simulink model "VC_v1p1"  (R2022b)
settings: Solver=VariableStepAuto  StartTime=0.0  StopTime=inf  FixedStep=1/100  MaxStep=ts  RelTol=1e-3
InitFcn:
  | init_car
  | init_par
values from neighbouring files (symbols this model uses):
  east0 = EWP(1)    [run_VC_bench.m]
  g = 9.81    [init_car.m]
  north0 = NWP(1)    [run_VC_bench.m]
  NUM_WP = length(NWP)    [run_VC_bench.m]
  psi0 = (pi/180)*HWP(1)    [run_VC_bench.m]
  ts = 1/fs    (= 0.01)    [init_car.m]
  vcg0 = 0    [run_VC_bench.m]
  WPT_MTX = [NWP,EWP,HWP,VWP,KWP,SWP]    [run_VC_bench.m]
undefined symbols (not defined in the file or in its folder): car, EWP, NWP, par, ZWP
libraries: simulink x9, matrix_library x6
(part 2 of 3)

== system VC_v1p1/Chevy Bolt EUV 2023 and GNSS/GNSS measurement/Project vc onto x-y axis ==
  psi (rad) : Inport
  vcg (m/s) : Inport  Port=2
  Product : Product  OutDataTypeStr=double
  Product1 : Product  OutDataTypeStr=double
  Trigonometric Function : Trigonometry  OutputSignalType=real
  Trigonometric Function1 : Trigonometry  Operator=cos  OutputSignalType=real
  vcgx (m/s) : Outport
  vcgy (m/s) : Outport  Port=2
  wires:
  Product/1 -> vcgx (m/s)/1  "vcgx (m/s)"
  Product1/1 -> vcgy (m/s)/1  "vcgy (m/s)"
  psi (rad)/1 -> Trigonometric Function1/1, Trigonometric Function/1
  Trigonometric Function1/1 -> Product/1
  Trigonometric Function/1 -> Product1/2
  vcg (m/s)/1 -> Product1/1, Product/2

== system VC_v1p1/Chevy Bolt EUV 2023 and GNSS/GNSS measurement/Subsystem ==
  note: $a_{lat} = \left( \frac{V_{cg}^2}{R} \right) = \left( \kappa\:V_{cg}^2 \right)$
  vcg (m/s) : Inport
  kappa (1/m) : Inport  Port=2
  multiply : Product
  multiply1 : Product
  alat (m/s/s) : Outport
  wires:
  vcg (m/s)/1 -> multiply/2, multiply/1
  kappa (1/m)/1 -> multiply1/2  "kappa (1/m)"
  multiply/1 -> multiply1/1  "vcg^2 (m^2/s^2)"
  multiply1/1 -> alat (m/s/s)/1  "alat (m/s/s)"

== system VC_v1p1/Chevy Bolt EUV 2023 and GNSS/engine-steer-brake and inertial dynamics/Brake Dynamics ==
  brake_cmd (Nm) : Inport
  torque_cmd (Nm) : Inport  Port=2
  Brake Saturation : Saturate  UpperLimit=car.MAX_BRAKE  LowerLimit=car.MIN_BRAKE  OutDataTypeStr=double
  Compare To Zero : simulink/Logic and Bit Operations/Compare To Zero  relop=>  OutDataTypeStr=boolean
  Compare To Zero1 : simulink/Logic and Bit Operations/Compare To Zero  relop=>=  OutDataTypeStr=boolean
  Logical Operator : Logic  Operator=OR  AllPortsSameDT=off  OutDataTypeStr=boolean
  Resettable Subsystem : Subsystem  TreatAsAtomicUnit=on
  brake dead zone : Subsystem
  brake_fbk (Nm) : Outport
  wires:
  brake_cmd (Nm)/1 -> Compare To Zero1/1, Brake Saturation/1
  Brake Saturation/1 -> Resettable Subsystem/1(In1)
  Resettable Subsystem/1(Out1) -> brake dead zone/1(brake_fbk)
  brake dead zone/1(brake_fbk (Nm)) -> brake_fbk (Nm)/1  "brake_fbk (Nm)"
  torque_cmd (Nm)/1 -> Compare To Zero/1
  Compare To Zero1/1 -> Logical Operator/2
  Compare To Zero/1 -> Logical Operator/1
  Logical Operator/1 -> Resettable Subsystem/Reset

== system VC_v1p1/Chevy Bolt EUV 2023 and GNSS/engine-steer-brake and inertial dynamics/Car Longitudinal Dynamics ==
  note: Note: vcg is the velocity measured at the CG of the car
  Fnet (N) : Inport
  1/ vehicle mass (kg) : Gain  Gain=1/car.MCAR  OutDataTypeStr=double
  Integrator : Integrator  InitialConditionSource=external
  initial vcg (m/s) : Constant  Value=vcg0
  velocity dead zone : Subsystem
  vcg (m/s) : Outport
  along  (m/s/s) : Outport  Port=2
  wires:
  1/ vehicle mass (kg)/1 -> along  (m/s/s)/1, Integrator/1  "acar (m/s/s)"
  Integrator/1 -> velocity dead zone/1(vcg)
  Fnet (N)/1 -> 1/ vehicle mass (kg)/1  "Fnet (N)"
  initial vcg (m/s)/1 -> Integrator/2
  velocity dead zone/1(vcg (m/s)) -> vcg (m/s)/1  "vcg (m/s)"

== system VC_v1p1/Chevy Bolt EUV 2023 and GNSS/engine-steer-brake and inertial dynamics/Engine Torque Dynamics ==
  note: gear: 1=drive, 0=park, -1=reverse
  torque_cmd (Nm) : Inport
  brake_cmd (Nm) : Inport  Port=2
  gear : Inport  Port=3
  Compare To Zero : simulink/Logic and Bit Operations/Compare To Zero  relop=<  OutDataTypeStr=boolean
  Compare To Zero1 : simulink/Logic and Bit Operations/Compare To Zero  relop=<=  OutDataTypeStr=boolean
  Constant : Constant  Value=0
  Constant1 : Constant  Value=0
  Logical Operator : Logic  Operator=OR  AllPortsSameDT=off  OutDataTypeStr=boolean
  Resettable Subsystem : Subsystem  TreatAsAtomicUnit=on
  Torque Saturation : Saturate  UpperLimit=car.MAX_TORQUE  LowerLimit=car.MIN_TORQUE  OutDataTypeStr=double
  do not allow any torque when in park : Switch  Criteria=u2 ~= 0  SaturateOnIntegerOverflow=off  InputSameDT=off
  "do not allow any torque when in park " : Switch  Criteria=u2 ~= 0  SaturateOnIntegerOverflow=off  InputSameDT=off
  torque dead zone : Subsystem
  torque_fbk (Nm) : Outport
  wires:
  gear/1 -> "do not allow any torque when in park "/2, do not allow any torque when in park/2
  torque_cmd (Nm)/1 -> Compare To Zero1/1, do not allow any torque when in park/1
  Constant/1 -> do not allow any torque when in park/3
  do not allow any torque when in park/1 -> Torque Saturation/1
  Constant1/1 -> "do not allow any torque when in park "/3
  "do not allow any torque when in park "/1 -> torque dead zone/1(torque_fbk)
  torque dead zone/1(torque_fbk (Nm)) -> torque_fbk (Nm)/1
  Torque Saturation/1 -> Resettable Subsystem/1(In1)
  Resettable Subsystem/1(Out1) -> "do not allow any torque when in park "/1  "torque_fbk (Nm)"
  brake_cmd (Nm)/1 -> Compare To Zero/1
  Logical Operator/1 -> Resettable Subsystem/Reset
  Compare To Zero/1 -> Logical Operator/1
  Compare To Zero1/1 -> Logical Operator/2

== system VC_v1p1/Chevy Bolt EUV 2023 and GNSS/engine-steer-brake and inertial dynamics/Net Force Applied at CG ==
  torque_fbk (Nm) : Inport
  brake_fbk (Nm) : Inport  Port=2
  Fgrade (N) : Inport  Port=3
  vcg (m/s) : Inport  Port=4
  1 / Tire Radius : Gain  Gain=1 / car.Rtire
  "1 / Tire Radius " : Gain  Gain=1 / car.Rtire
  Bus Creator : BusCreator  Inputs=4
  MATLAB Function : MATLAB Function  TreatAsAtomicUnit=on
  Sum : Sum  Inputs=++-
  To Workspace2 : ToWorkspace  VariableName=forces  SampleTime=ts
  deadzone velocity1 : Constant  Value=car.Vdead  SampleTime=ts
  rolling resistance (Ns/m) : Gain  Gain=car.RRdamp
  Fnet (N) : Outport
  wires:
  vcg (m/s)/1 -> MATLAB Function/3(vcg), rolling resistance (Ns/m)/1
  torque_fbk (Nm)/1 -> 1 / Tire Radius/1
  brake_fbk (Nm)/1 -> "1 / Tire Radius "/1
  1 / Tire Radius/1 -> Sum/2  "Ftorque (N)"
  "1 / Tire Radius "/1 -> MATLAB Function/4(Fbrake)  "Fbrake (N)"
  deadzone velocity1/1 -> MATLAB Function/2(Vdead)
  rolling resistance (Ns/m)/1 -> Bus Creator/4, Sum/3  "Fdamp (N)"
  Sum/1 -> Bus Creator/2, MATLAB Function/1(Fsum)  "Fsum (N)"
  Fgrade (N)/1 -> Bus Creator/1, Sum/1  "Fgrade (N)"
  Bus Creator/1 -> To Workspace2/1
  MATLAB Function/1(Fnet) -> Bus Creator/3, Fnet (N)/1  "Fnet (N)"

== system VC_v1p1/Chevy Bolt EUV 2023 and GNSS/engine-steer-brake and inertial dynamics/Road Grade Force ==
  note: NOTE: Positive grade (pitch) means "pointing uphill", which makes the force due to grade (Fgrade) have a negative value as well as the resulting effective grade torque (Tgrade).
  grade (rad) : Inport
  gear_fbk : Inport  Port=2
  Compare To Zero : simulink/Logic and Bit Operations/Compare To Zero  relop=~=  OutDataTypeStr=boolean
  Constant : Constant  Value=0
  Do not allow grade force when car is in Park : Switch  Criteria=u2 > Threshold  SaturateOnIntegerOverflow=off  InputSameDT=off
  To Workspace2 : ToWorkspace  VariableName=Fgrade  SampleTime=ts
  Trigonometric Function : Trigonometry
  account for direction of force with grade : Gain  Gain=-1
  grade component : Gain  Gain=car.MCAR * g  OutDataTypeStr=double
  pitch (rad) : Outport
  Fgrade (N) : Outport  Port=2
  wires:
  grade component/1 -> account for direction of force with grade/1
  grade (rad)/1 -> pitch (rad)/1, Trigonometric Function/1  "assume no pitch dynamics so pitch = grade"
  Trigonometric Function/1 -> grade component/1
  account for direction of force with grade/1 -> Do not allow grade force when car is in Park/1
  Compare To Zero/1 -> Do not allow grade force when car is in Park/2
  gear_fbk/1 -> Compare To Zero/1
  Constant/1 -> Do not allow grade force when car is in Park/3
  Do not allow grade force when car is in Park/1 -> To Workspace2/1, Fgrade (N)/1  "Fgrade (Nm)"

== system VC_v1p1/Chevy Bolt EUV 2023 and GNSS/engine-steer-brake and inertial dynamics/Steering Dynamics ==
  steer_cmd (deg) : Inport
  Gain conversion from steering angle (deg) to front wheel angle (deg) : Gain  Gain=car.STEER_RATIO
  Steering Saturation : Saturate  UpperLimit=car.MAX_STEER  LowerLimit=car.MIN_STEER  OutDataTypeStr=double
  deg-to-rad : Gain  Gain=pi/180
  second-order low-pass steer model : TransferFcn  Numerator=car.STEER_NUMS  Denominator=car.STEER_DENS
  steer dead zone : Subsystem
  delta (rad) : Outport
  steer_fbk (deg) : Outport  Port=2
  wires:
  Steering Saturation/1 -> second-order low-pass steer model/1
  steer_cmd (deg)/1 -> Steering Saturation/1
  Gain conversion from steering angle (deg) to front wheel angle (deg)/1 -> deg-to-rad/1  "front wheel  angle (deg)"
  deg-to-rad/1 -> delta (rad)/1
  second-order low-pass steer model/1 -> steer dead zone/1(steer)
  steer dead zone/1(steer (deg)) -> steer_fbk (deg)/1, Gain conversion from steering angle (deg) to front wheel angle (deg)/1  "actual steering wheel angle (deg)"

== system VC_v1p1/Chevy Bolt EUV 2023 and GNSS/kinematic Bicycle model/CG to Rear Coordinate Transformation ==
  pose_cg : Inport
  beta : Inport  Port=2
  Bus Creator1 : BusCreator  Inputs=4
  Bus Selector : BusSelector  OutputSignals=eastcg (m),psi (rad),northcg (m),vcg (m/s)
  Product4 : Product
  Sum7 : Sum  Inputs=+-|
  Sum8 : Sum  Inputs=|-+
  Trigonometric Function5 : Trigonometry  Operator=cos  OutputSignalType=real
  Trigonometric Function6 : Trigonometry  OutputSignalType=real
  Trigonometric Function7 : Trigonometry  Operator=cos  OutputSignalType=real
  cg to rear wheel (m) : Gain  Gain=car.LR
  cg to rear wheel (m)2 : Gain  Gain=car.LR
  pose_rear : Outport
  wires:
  Trigonometric Function6/1 -> cg to rear wheel (m)/1
  Bus Selector/1 -> Sum7/1  "<eastcg (m)>"
  cg to rear wheel (m)/1 -> Sum7/2
  Bus Selector/2 -> Trigonometric Function6/1, Bus Creator1/3, Trigonometric Function5/1  "<psi (rad)>"
  Trigonometric Function5/1 -> cg to rear wheel (m)2/1
  Sum8/1 -> Bus Creator1/2  "northr (m)"
  cg to rear wheel (m)2/1 -> Sum8/1
  Bus Creator1/1 -> pose_rear/1
  beta/1 -> Trigonometric Function7/1
  pose_cg/1 -> Bus Selector/1
  Sum7/1 -> Bus Creator1/1  "eastr (m)"
  Bus Selector/3 -> Sum8/2  "<northcg (m)>"
  Trigonometric Function7/1 -> Product4/2
  Bus Selector/4 -> Product4/1  "<vcg (m/s)>"
  Product4/1 -> Bus Creator1/4  "vr (m/s)"

== system VC_v1p1/Chevy Bolt EUV 2023 and GNSS/kinematic Bicycle model/Vehicle Slip Angle (direction of CG) ==
  note: Curvature: $\kappa = \left( \frac{1}{radius\:of\:curvature} \right)$
  note: Equation 2.7, pg. 23, Rajamani
  note: Equation 2.13, pg. 24, Rajamani
  note: $\beta$ = slip angle of vehicle [radians]
  delta (rad) : Inport
  Divide : Product  Inputs=**/
  Trigonometric Function1 : Trigonometry  Operator=cos  OutputSignalType=real
  Trigonometric Function2 : Trigonometry  Operator=atan2  OutputSignalType=real
  Trigonometric Function3 : Trigonometry  Operator=tan  OutputSignalType=real
  cg to rear wheel (m) : Gain  Gain=car.LR
  wheelbase (m) : Constant  Value=car.LF+car.LR
  "wheelbase (m) " : Constant  Value=car.LF+car.LR
  beta (rad) : Outport
  kappa (1/m) : Outport  Port=2
  wires:
  wheelbase (m)/1 -> Trigonometric Function2/2
  Trigonometric Function2/1 -> Trigonometric Function1/1, beta (rad)/1  "beta"
  Trigonometric Function3/1 -> Divide/2, cg to rear wheel (m)/1  "tan(delta)"
  delta (rad)/1 -> Trigonometric Function3/1
  cg to rear wheel (m)/1 -> Trigonometric Function2/1
  Trigonometric Function1/1 -> Divide/1
  "wheelbase (m) "/1 -> Divide/3
  Divide/1 -> kappa (1/m)/1  "1/R"

== system VC_v1p1/Vehicle_Controller/Data Registers/load new parameter vector ==
  mode_select : Inport
  par_vector : Inport  Port=2
  Subsystem : Subsystem
  edge detector : Subsystem
  par_bus_out : Outport
  wires:
  mode_select/1 -> edge detector/1(in)
  par_vector/1 -> Subsystem/1(par_vector)
  Subsystem/1(par_bus) -> par_bus_out/1
  edge detector/1(out) -> Subsystem/Enable

== system VC_v1p1/Vehicle_Controller/Data Registers/load new waypoint matrix ==
  new_wpts : Inport
  num_wp : Inport  Port=2
  wpt_mtx : Inport  Port=3
  Data Type Conversion : DataTypeConversion  OutDataTypeStr=double  SaturateOnIntegerOverflow=off  RndMeth=Floor
  Subsystem : Subsystem
  edge detector : Subsystem
  wpt_status_change : Outport
  wpt_bus_out : Outport  Port=2
  wires:
  wpt_mtx/1 -> Subsystem/2(WPT_MTX)
  new_wpts/1 -> edge detector/1(in)
  edge detector/1(out) -> Data Type Conversion/1, Subsystem/Enable
  Data Type Conversion/1 -> wpt_status_change/1
  Subsystem/1(WPT_BUS) -> wpt_bus_out/1
  num_wp/1 -> Subsystem/1(NUM_WP)

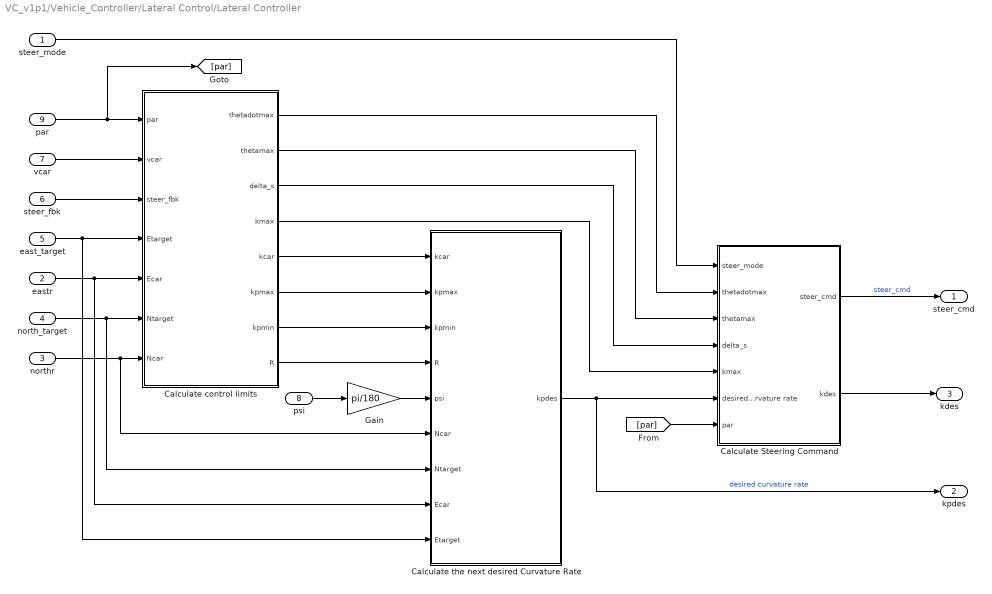
== system VC_v1p1/Vehicle_Controller/Lateral Control/Lateral Controller ==
  steer_mode : Inport
  eastr : Inport  Port=2
  northr : Inport  Port=3
  north_target : Inport  Port=4
  east_target : Inport  Port=5
  steer_fbk : Inport  Port=6
  vcar : Inport  Port=7
  psi : Inport  Port=8
  par : Inport  Port=9
  Calculate Steering Command : Subsystem
  Calculate control limits : Subsystem
  Calculate the next desired Curvature Rate : MATLAB Function  TreatAsAtomicUnit=on  SystemSampleTime=ts
  Gain : Gain  Gain=pi/180
  steer_cmd : Outport
  kpdes : Outport  Port=2
  kdes : Outport  Port=3
  wires:
  par/1 -> [par], Calculate control limits/1(par)
  psi/1 -> Gain/1
  vcar/1 -> Calculate control limits/2(vcar)
  steer_fbk/1 -> Calculate control limits/3(steer_fbk)
  Calculate control limits/5(kcar) -> Calculate the next desired Curvature Rate/1(kcar)
  Calculate control limits/6(kpmax) -> Calculate the next desired Curvature Rate/2(kpmax)
  Calculate control limits/7(kpmin) -> Calculate the next desired Curvature Rate/3(kpmin)
  Calculate control limits/8(R) -> Calculate the next desired Curvature Rate/4(R)
  east_target/1 -> Calculate the next desired Curvature Rate/9(Etarget), Calculate control limits/4(Etarget)
  eastr/1 -> Calculate the next desired Curvature Rate/8(Ecar), Calculate control limits/5(Ecar)
  north_target/1 -> Calculate the next desired Curvature Rate/7(Ntarget), Calculate control limits/6(Ntarget)
  northr/1 -> Calculate the next desired Curvature Rate/6(Ncar), Calculate control limits/7(Ncar)
  steer_mode/1 -> Calculate Steering Command/1(steer_mode)
  Calculate control limits/1(thetadotmax) -> Calculate Steering Command/2(thetadotmax)
  Calculate control limits/2(thetamax) -> Calculate Steering Command/3(thetamax)
  Calculate control limits/3(delta_s) -> Calculate Steering Command/4(delta_s)
  Calculate control limits/4(kmax) -> Calculate Steering Command/5(kmax)
  Calculate the next desired Curvature Rate/1(kpdes) -> kpdes/1, Calculate Steering Command/6(desired curvature rate)  "desired curvature rate"
  [par] -> Calculate Steering Command/7(par)
  Calculate Steering Command/1(steer_cmd) -> steer_cmd/1  "steer_cmd"
  Gain/1 -> Calculate the next desired Curvature Rate/5(psi)
  Calculate Steering Command/2(kdes) -> kdes/1

== system VC_v1p1/Vehicle_Controller/Longitudinal Control/Longitudinal Controller ==
  speed_mode : Inport
  vref : Inport  Port=2
  vcar : Inport  Port=3
  alat : Inport  Port=4
  along : Inport  Port=5
  pitch : Inport  Port=6
  par : Inport  Port=7
  Speed Controller : Subsystem
  velocity feedback pre-processor : Subsystem
  torque_cmd : Outport
  brake_cmd : Outport  Port=2
  vdes : Outport  Port=3
  car_is_stopped : Outport  Port=4
  wires:
  velocity feedback pre-processor/3(verror) -> Speed Controller/2(verror)
  speed_mode/1 -> velocity feedback pre-processor/1(speed_mode), Speed Controller/1(speed_mode)
  par/1 -> Speed Controller/4(par), velocity feedback pre-processor/6(par)
  alat/1 -> velocity feedback pre-processor/4(alat)
  vref/1 -> velocity feedback pre-processor/2(vref)
  velocity feedback pre-processor/1(vdes) -> vdes/1
  vcar/1 -> velocity feedback pre-processor/3(vcar)
  along/1 -> velocity feedback pre-processor/5(along)
  pitch/1 -> Speed Controller/3(pitch)
  Speed Controller/1(torque_cmd) -> torque_cmd/1
  Speed Controller/2(brake_cmd) -> brake_cmd/1
  velocity feedback pre-processor/2(car_is_stopped) -> car_is_stopped/1

== system VC_v1p1/Vehicle_Controller/Pack Data Log Message/Estimate Jerk ==
  Bus Selector : BusSelector  OutputSignals=ts
  Jerk Estimation Filter : MATLAB Function  TreatAsAtomicUnit=on  SystemSampleTime=ts
  jlat (m/s/s/s) : Outport
  jlong (m/s/s/s) : Outport  Port=2
  wires:
  Jerk Estimation Filter/1(jlat) -> jlat (m/s/s/s)/1  "jlat (m/s/s/s)"
  Jerk Estimation Filter/2(jlong) -> jlong (m/s/s/s)/1  "jlong (m/s/s/s)"
  [alat] -> Jerk Estimation Filter/2(alat)
  [along] -> Jerk Estimation Filter/3(along)
  [mode_select] -> Jerk Estimation Filter/1(mode_select)
  [par_bus] -> Bus Selector/1
  Bus Selector/1 -> Jerk Estimation Filter/4(ts)  "<ts>"

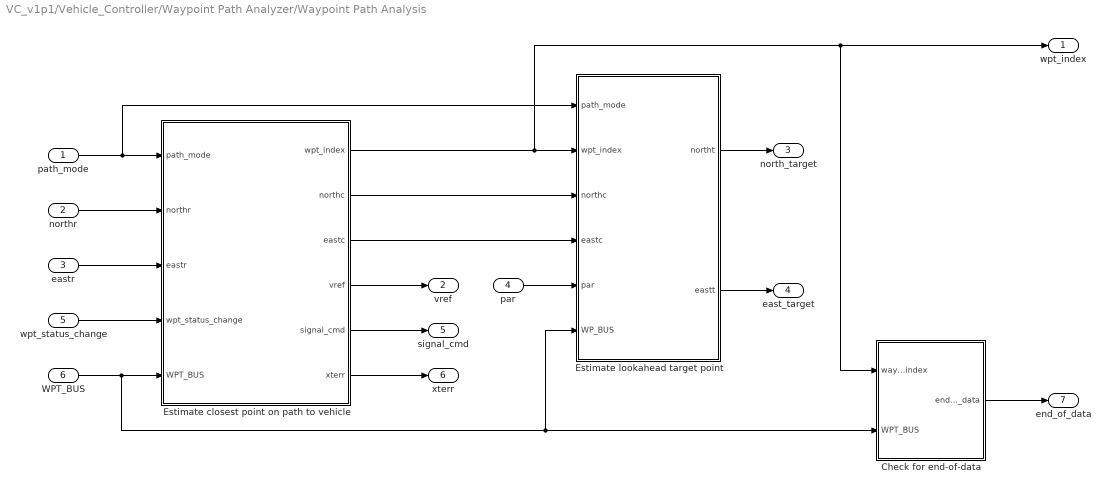
== system VC_v1p1/Vehicle_Controller/Waypoint Path Analyzer/Waypoint Path Analysis ==
  path_mode : Inport
  northr : Inport  Port=2
  eastr : Inport  Port=3
  par : Inport  Port=4
  wpt_status_change : Inport  Port=5
  WPT_BUS : Inport  Port=6
  Check for end-of-data : Subsystem
  Estimate closest point on path to vehicle : Subsystem
  Estimate lookahead target point : Subsystem
  wpt_index : Outport
  vref : Outport  Port=2
  north_target : Outport  Port=3
  east_target : Outport  Port=4
  signal_cmd : Outport  Port=5
  xterr : Outport  Port=6
  end_of_data : Outport  Port=7
  wires:
  path_mode/1 -> Estimate lookahead target point/1(path_mode), Estimate closest point on path to vehicle/1(path_mode)
  Estimate closest point on path to vehicle/2(northc) -> Estimate lookahead target point/3(northc)
  Estimate closest point on path to vehicle/3(eastc) -> Estimate lookahead target point/4(eastc)
  Estimate closest point on path to vehicle/1(wpt_index) -> Check for end-of-data/1(waypoint_index), wpt_index/1, Estimate lookahead target point/2(wpt_index)
  wpt_status_change/1 -> Estimate closest point on path to vehicle/4(wpt_status_change)
  WPT_BUS/1 -> Estimate lookahead target point/6(WP_BUS), Check for end-of-data/2(WPT_BUS), Estimate closest point on path to vehicle/5(WPT_BUS)
  par/1 -> Estimate lookahead target point/5(par)
  Estimate lookahead target point/1(northt) -> north_target/1
  Estimate lookahead target point/2(eastt) -> east_target/1
  Estimate closest point on path to vehicle/4(vref) -> vref/1
  Estimate closest point on path to vehicle/5(signal_cmd) -> signal_cmd/1
  Estimate closest point on path to vehicle/6(xterr) -> xterr/1
  Check for end-of-data/1(end_of_data) -> end_of_data/1
  northr/1 -> Estimate closest point on path to vehicle/2(northr)
  eastr/1 -> Estimate closest point on path to vehicle/3(eastr)

== system VC_v1p1/Chevy Bolt EUV 2023 and GNSS/engine-steer-brake and inertial dynamics/Brake Dynamics/Resettable Subsystem ==
  In1 : Inport
  Reset : ResetPort  DisableCoverage=on
  second-order low-pass brake model : TransferFcn  Numerator=car.BRAKE_NUMS  Denominator=car.BRAKE_DENS
  Out1 : Outport
  wires:
  In1/1 -> second-order low-pass brake model/1
  second-order low-pass brake model/1 -> Out1/1  "brake_fbk (Nm)"

== system VC_v1p1/Chevy Bolt EUV 2023 and GNSS/engine-steer-brake and inertial dynamics/Brake Dynamics/brake dead zone ==
  brake_fbk : Inport
  Abs : Abs  SaturateOnIntegerOverflow=off
  Compare To Constant : simulink/Logic and Bit Operations/Compare To Constant  relop=>  const=car.Tdead  OutDataTypeStr=boolean
  Constant2 : Constant  Value=0
  Zero output signal when in dead zone : Switch  Criteria=u2 > Threshold  SaturateOnIntegerOverflow=off  InputSameDT=off
  brake_fbk (Nm) : Outport
  wires:
  brake_fbk/1 -> Abs/1, Zero output signal when in dead zone/1
  Abs/1 -> Compare To Constant/1
  Zero output signal when in dead zone/1 -> brake_fbk (Nm)/1  "brake_fbk (Nm)"
  Compare To Constant/1 -> Zero output signal when in dead zone/2
  Constant2/1 -> Zero output signal when in dead zone/3

== system VC_v1p1/Chevy Bolt EUV 2023 and GNSS/engine-steer-brake and inertial dynamics/Car Longitudinal Dynamics/velocity dead zone ==
  vcg : Inport
  Abs : Abs  SaturateOnIntegerOverflow=off
  Compare To Constant : simulink/Logic and Bit Operations/Compare To Constant  relop=>  const=car.Vdead  OutDataTypeStr=boolean
  Constant2 : Constant  Value=0
  Zero output signal when in dead zone : Switch  Criteria=u2 > Threshold  SaturateOnIntegerOverflow=off  InputSameDT=off
  vcg (m/s) : Outport
  wires:
  vcg/1 -> Abs/1, Zero output signal when in dead zone/1
  Abs/1 -> Compare To Constant/1
  Zero output signal when in dead zone/1 -> vcg (m/s)/1  "vcg (m/s)"
  Compare To Constant/1 -> Zero output signal when in dead zone/2
  Constant2/1 -> Zero output signal when in dead zone/3

== system VC_v1p1/Chevy Bolt EUV 2023 and GNSS/engine-steer-brake and inertial dynamics/Engine Torque Dynamics/Resettable Subsystem ==
  In1 : Inport
  Reset : ResetPort  DisableCoverage=on
  second-order low-pass torque model : TransferFcn  Numerator=car.TORQUE_NUMS  Denominator=car.TORQUE_DENS
  Out1 : Outport
  wires:
  In1/1 -> second-order low-pass torque model/1
  second-order low-pass torque model/1 -> Out1/1  "torque_fbk (Nm)"

== system VC_v1p1/Chevy Bolt EUV 2023 and GNSS/engine-steer-brake and inertial dynamics/Engine Torque Dynamics/torque dead zone ==
  torque_fbk : Inport
  Abs : Abs  SaturateOnIntegerOverflow=off
  Compare To Constant : simulink/Logic and Bit Operations/Compare To Constant  relop=>  const=car.Tdead  OutDataTypeStr=boolean
  Constant2 : Constant  Value=0
  Zero output signal when in dead zone : Switch  Criteria=u2 > Threshold  SaturateOnIntegerOverflow=off  InputSameDT=off
  torque_fbk (Nm) : Outport
  wires:
  torque_fbk/1 -> Abs/1, Zero output signal when in dead zone/1
  Abs/1 -> Compare To Constant/1
  Zero output signal when in dead zone/1 -> torque_fbk (Nm)/1  "torque_fbk (Nm)"
  Compare To Constant/1 -> Zero output signal when in dead zone/2
  Constant2/1 -> Zero output signal when in dead zone/3

== system VC_v1p1/Chevy Bolt EUV 2023 and GNSS/engine-steer-brake and inertial dynamics/Steering Dynamics/steer dead zone ==
  steer : Inport
  Abs : Abs  SaturateOnIntegerOverflow=off
  Compare To Constant : simulink/Logic and Bit Operations/Compare To Constant  relop=>  const=0.5  OutDataTypeStr=boolean
  Constant2 : Constant  Value=0
  Zero output signal when in dead zone : Switch  Criteria=u2 > Threshold  SaturateOnIntegerOverflow=off  InputSameDT=off
  steer (deg) : Outport
  wires:
  steer/1 -> Abs/1, Zero output signal when in dead zone/1
  Abs/1 -> Compare To Constant/1
  Zero output signal when in dead zone/1 -> steer (deg)/1  "steer (deg)"
  Compare To Constant/1 -> Zero output signal when in dead zone/2
  Constant2/1 -> Zero output signal when in dead zone/3

== system VC_v1p1/Vehicle_Controller/Data Registers/load new parameter vector/Subsystem ==
  note: Initialize par_bus with a default vcctor of values. Whenever this subsystem is enabled, a new par_vector is pushed into the par_bus.
      |
      | The output values stored in par_bus are latched when this subsystem is disabled.
  par_vector : Inport
  Enable : EnablePort  ShowOutputPort=on
  Bus Creator : BusCreator  Inputs=32
  Demux : Demux  Outputs=32
  Initial Control Parameters : Constant  Value=par  SampleTime=ts
  Switch : Switch  Criteria=u2 > Threshold  SaturateOnIntegerOverflow=off  InputSameDT=off
  par_bus : Outport
  wires:
  Demux/26 -> Bus Creator/26  "min_lookahead"
  Demux/29 -> Bus Creator/29  "wT"
  Demux/12 -> Bus Creator/12  "min_steer"
  Demux/1 -> Bus Creator/1  "ts"
  Demux/32 -> Bus Creator/32  "zB"
  Demux/27 -> Bus Creator/27  "lookahead_ratelimit"
  Demux/10 -> Bus Creator/10  "max_alat"
  Demux/31 -> Bus Creator/31  "wB"
  Demux/14 -> Bus Creator/14  "kp_speed"
  Demux/24 -> Bus Creator/24  "fbreak_vref"
  Demux/7 -> Bus Creator/7  "max_delta_brake"
  Demux/21 -> Bus Creator/21  "zz_lead"
  Demux/25 -> Bus Creator/25  "max_lookahead"
  Demux/13 -> Bus Creator/13  "max_delta_steer"
  Demux/17 -> Bus Creator/17  "fbreak_diff"
  Demux/8 -> Bus Creator/8  "max_speed"
  Demux/18 -> Bus Creator/18  "kff_gain"
  Demux/20 -> Bus Creator/20  "fz_lead"
  Demux/28 -> Bus Creator/28  "vdead"
  Demux/15 -> Bus Creator/15  "ki_speed"
  Demux/22 -> Bus Creator/22  "fp_lead"
  Demux/3 -> Bus Creator/3  "min_drv_torque"
  Demux/30 -> Bus Creator/30  "zT"
  Demux/16 -> Bus Creator/16  "kd_speed"
  Demux/9 -> Bus Creator/9  "min_speed"
  Demux/23 -> Bus Creator/23  "kappa2theta"
  Bus Creator/1 -> par_bus/1
  Demux/19 -> Bus Creator/19  "fbreak_fflpf"
  Demux/6 -> Bus Creator/6  "max_delta_torque"
  Demux/4 -> Bus Creator/4  "max_brk_torque"
  Demux/11 -> Bus Creator/11  "max_steer"
  Demux/5 -> Bus Creator/5  "min_brk_torque"
  Demux/2 -> Bus Creator/2  "max_drv_torque"
  par_vector/1 -> Switch/1
  Enable/1 -> Switch/2
  Initial Control Parameters/1 -> Switch/3
  Switch/1 -> Demux/1

== system VC_v1p1/Vehicle_Controller/Data Registers/load new parameter vector/edge detector ==
  note: edge detector
  in : Inport
  Relational Operator : RelationalOperator  Operator=~=  OutDataTypeStr=boolean  RndMeth=Simplest  InputSameDT=off
  previous in : UnitDelay  InitialCondition=3  SampleTime=ts  HasFrameUpgradeWarning=on
  out : Outport
  wires:
  in/1 -> Relational Operator/1, previous in/1
  previous in/1 -> Relational Operator/2
  Relational Operator/1 -> out/1

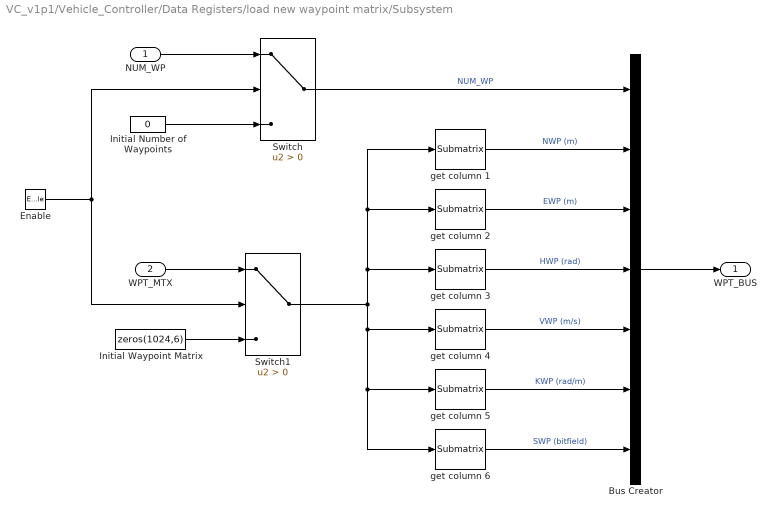
== system VC_v1p1/Vehicle_Controller/Data Registers/load new waypoint matrix/Subsystem ==
  NUM_WP : Inport
  WPT_MTX : Inport  Port=2
  Enable : EnablePort  ShowOutputPort=on
  Bus Creator : BusCreator  Inputs=7
  Initial Waypoint Matrix : Constant  Value=zeros(1024,6)  SampleTime=ts
  "Initial Number of Waypoints   " : Constant  Value=0  SampleTime=ts
  Switch : Switch  Criteria=u2 > Threshold  SaturateOnIntegerOverflow=off  InputSameDT=off
  Switch1 : Switch  Criteria=u2 > Threshold  SaturateOnIntegerOverflow=off  InputSameDT=off
  get column 1 : matrix_library/Submatrix  RowSpan=All rows  RowStartMode=First  RowStartIndex=1  RowEndMode=Last  RowEndIndex=1  ColSpan=One column  ColStartMode=Index  ColStartIndex=1  ColEndMode=Last  ColEndIndex=1
  get column 2 : matrix_library/Submatrix  RowSpan=All rows  RowStartMode=First  RowStartIndex=1  RowEndMode=Last  RowEndIndex=1  ColSpan=One column  ColStartMode=Index  ColStartIndex=2  ColEndMode=Last  ColEndIndex=1
  get column 3 : matrix_library/Submatrix  RowSpan=All rows  RowStartMode=First  RowStartIndex=1  RowEndMode=Last  RowEndIndex=1  ColSpan=One column  ColStartMode=Index  ColStartIndex=3  ColEndMode=Last  ColEndIndex=1
  get column 4 : matrix_library/Submatrix  RowSpan=All rows  RowStartMode=First  RowStartIndex=1  RowEndMode=Last  RowEndIndex=1  ColSpan=One column  ColStartMode=Index  ColStartIndex=4  ColEndMode=Last  ColEndIndex=1
  get column 5 : matrix_library/Submatrix  RowSpan=All rows  RowStartMode=First  RowStartIndex=1  RowEndMode=Last  RowEndIndex=1  ColSpan=One column  ColStartMode=Index  ColStartIndex=5  ColEndMode=Last  ColEndIndex=1
  get column 6 : matrix_library/Submatrix  RowSpan=All rows  RowStartMode=First  RowStartIndex=1  RowEndMode=Last  RowEndIndex=1  ColSpan=One column  ColStartMode=Index  ColStartIndex=6  ColEndMode=Last  ColEndIndex=1
  WPT_BUS : Outport
  wires:
  Bus Creator/1 -> WPT_BUS/1
  get column 4/1 -> Bus Creator/5  "VWP (m/s)"
  get column 5/1 -> Bus Creator/6  "KWP (rad/m)"
  get column 1/1 -> Bus Creator/2  "NWP (m)"
  get column 3/1 -> Bus Creator/4  "HWP (rad)"
  get column 2/1 -> Bus Creator/3  "EWP (m)"
  get column 6/1 -> Bus Creator/7  "SWP (bitfield)"
  Switch/1 -> Bus Creator/1  "NUM_WP"
  NUM_WP/1 -> Switch/1
  WPT_MTX/1 -> Switch1/1
  Switch1/1 -> get column 6/1, get column 5/1, get column 4/1, get column 3/1, get column 2/1, get column 1/1
  Enable/1 -> Switch/2, Switch1/2
  "Initial Number of Waypoints   "/1 -> Switch/3
  Initial Waypoint Matrix/1 -> Switch1/3

== system VC_v1p1/Vehicle_Controller/Data Registers/load new waypoint matrix/edge detector ==
  note: edge detector
  in : Inport
  Relational Operator : RelationalOperator  Operator=~=  OutDataTypeStr=boolean  RndMeth=Simplest  InputSameDT=off
  previous in : UnitDelay  SampleTime=ts  HasFrameUpgradeWarning=on
  out : Outport
  wires:
  in/1 -> Relational Operator/1, previous in/1
  previous in/1 -> Relational Operator/2
  Relational Operator/1 -> out/1

== system VC_v1p1/Vehicle_Controller/Lateral Control/Lateral Controller/Calculate Steering Command ==
  steer_mode : Inport
  thetadotmax : Inport  Port=2
  thetamax : Inport  Port=3
  delta_s : Inport  Port=4
  kmax : Inport  Port=5
  desired curvature rate : Inport  Port=6
  par : Inport  Port=7
  Bus Selector1 : BusSelector  OutputSignals=kappa2theta,ts,max_steer,min_steer,max_delta_steer
  Bus Selector2 : BusSelector  OutputSignals=ts,fz_lead,zz_lead,fp_lead
  Integrate Curvature Rate and compute next Steering Command : MATLAB Function  TreatAsAtomicUnit=on  SystemSampleTime=ts
  MATLAB Function : MATLAB Function  TreatAsAtomicUnit=on  SystemSampleTime=ts
  steer_cmd : Outport
  kdes : Outport  Port=2
  wires:
  desired curvature rate/1 -> Integrate Curvature Rate and compute next Steering Command/6(kpdes)
  thetadotmax/1 -> Integrate Curvature Rate and compute next Steering Command/2(thetadotmax)
  Bus Selector1/1 -> Integrate Curvature Rate and compute next Steering Command/7(kappa2theta)  "<kappa2theta>"
  delta_s/1 -> Integrate Curvature Rate and compute next Steering Command/4(delta_s)
  steer_mode/1 -> MATLAB Function/1(steer_mode), Integrate Curvature Rate and compute next Steering Command/1(steer_mode)
  par/1 -> Bus Selector2/1, Bus Selector1/1
  kmax/1 -> Integrate Curvature Rate and compute next Steering Command/5(kmax)
  Bus Selector1/3 -> Integrate Curvature Rate and compute next Steering Command/9(max_steer)  "<max_steer>"
  thetamax/1 -> Integrate Curvature Rate and compute next Steering Command/3(thetamax)
  Bus Selector1/4 -> Integrate Curvature Rate and compute next Steering Command/10(min_steer)  "<min_steer>"
  Bus Selector1/5 -> Integrate Curvature Rate and compute next Steering Command/11(max_delta_steer)  "<max_delta_steer>"
  Bus Selector1/2 -> Integrate Curvature Rate and compute next Steering Command/8(ts)  "<ts>"
  Integrate Curvature Rate and compute next Steering Command/1(steer_cmd) -> MATLAB Function/2(steer_cmd)
  MATLAB Function/1(steer_lead) -> steer_cmd/1
  Bus Selector2/1 -> MATLAB Function/3(ts)  "<ts>"
  Bus Selector2/2 -> MATLAB Function/4(fz_lead)  "<fz_lead>"
  Bus Selector2/3 -> MATLAB Function/5(zz_lead)  "<zz_lead>"
  Bus Selector2/4 -> MATLAB Function/6(fp_lead)  "<fp_lead>"
  Integrate Curvature Rate and compute next Steering Command/2(kdes) -> kdes/1

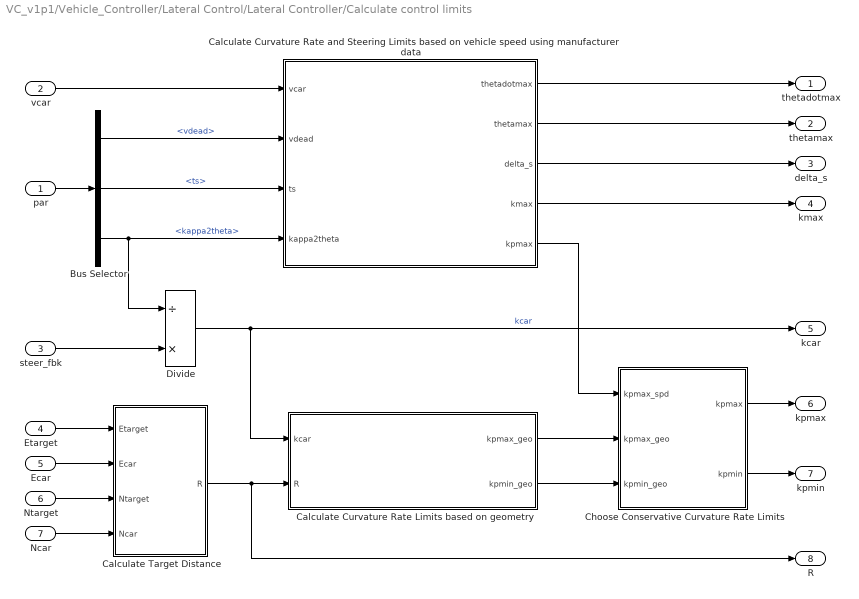
== system VC_v1p1/Vehicle_Controller/Lateral Control/Lateral Controller/Calculate control limits ==
  par : Inport
  vcar : Inport  Port=2
  steer_fbk : Inport  Port=3
  Etarget : Inport  Port=4
  Ecar : Inport  Port=5
  Ntarget : Inport  Port=6
  Ncar : Inport  Port=7
  Bus Selector : BusSelector  OutputSignals=vdead,ts,kappa2theta
  Calculate Curvature Rate Limits based on geometry : MATLAB Function  TreatAsAtomicUnit=on  SystemSampleTime=ts
  Calculate Curvature Rate and Steering Limits based on vehicle speed using manufacturer data : MATLAB Function  TreatAsAtomicUnit=on  SystemSampleTime=ts
  Calculate Target Distance : Subsystem
  Choose Conservative Curvature Rate Limits : Subsystem
  Divide : Product  Inputs=/*
  thetadotmax : Outport
  thetamax : Outport  Port=2
  delta_s : Outport  Port=3
  kmax : Outport  Port=4
  kcar : Outport  Port=5
  kpmax : Outport  Port=6
  kpmin : Outport  Port=7
  R : Outport  Port=8
  wires:
  Ntarget/1 -> Calculate Target Distance/3(Ntarget)
  Ecar/1 -> Calculate Target Distance/2(Ecar)
  Etarget/1 -> Calculate Target Distance/1(Etarget)
  Choose Conservative Curvature Rate Limits/1(kpmax) -> kpmax/1
  Calculate Curvature Rate Limits based on geometry/2(kpmin_geo) -> Choose Conservative Curvature Rate Limits/3(kpmin_geo)
  Ncar/1 -> Calculate Target Distance/4(Ncar)
  vcar/1 -> Calculate Curvature Rate and Steering Limits based on vehicle speed using manufacturer data/1(vcar)
  Calculate Curvature Rate Limits based on geometry/1(kpmax_geo) -> Choose Conservative Curvature Rate Limits/2(kpmax_geo)
  Choose Conservative Curvature Rate Limits/2(kpmin) -> kpmin/1
  steer_fbk/1 -> Divide/2
  Divide/1 -> Calculate Curvature Rate Limits based on geometry/1(kcar), kcar/1  "kcar"
  Calculate Target Distance/1(R) -> R/1, Calculate Curvature Rate Limits based on geometry/2(R)
  Calculate Curvature Rate and Steering Limits based on vehicle speed using manufacturer data/5(kpmax) -> Choose Conservative Curvature Rate Limits/1(kpmax_spd)
  Calculate Curvature Rate and Steering Limits based on vehicle speed using manufacturer data/4(kmax) -> kmax/1
  Calculate Curvature Rate and Steering Limits based on vehicle speed using manufacturer data/3(delta_s) -> delta_s/1
  Calculate Curvature Rate and Steering Limits based on vehicle speed using manufacturer data/1(thetadotmax) -> thetadotmax/1
  Calculate Curvature Rate and Steering Limits based on vehicle speed using manufacturer data/2(thetamax) -> thetamax/1
  par/1 -> Bus Selector/1
  Bus Selector/1 -> Calculate Curvature Rate and Steering Limits based on vehicle speed using manufacturer data/2(vdead)  "<vdead>"
  Bus Selector/2 -> Calculate Curvature Rate and Steering Limits based on vehicle speed using manufacturer data/3(ts)  "<ts>"
  Bus Selector/3 -> Divide/1, Calculate Curvature Rate and Steering Limits based on vehicle speed using manufacturer data/4(kappa2theta)  "<kappa2theta>"

== system VC_v1p1/Vehicle_Controller/Longitudinal Control/Longitudinal Controller/Speed Controller ==
  speed_mode : Inport
  verror : Inport  Port=2
  pitch : Inport  Port=3
  par : Inport  Port=4
  Bus Selector1 : BusSelector  OutputSignals=ts,max_drv_torque,max_delta_torque,min_brk_torque,max_delta_brake,kp_speed,ki_speed,kd_speed,kff_gain,fbreak_diff,fbreak_fflpf
  Bus Selector2 : BusSelector  OutputSignals=ts,wT,zT,wB,zB,min_brk_torque
  Compensate brake path : MATLAB Function  TreatAsAtomicUnit=on  SystemSampleTime=ts
  PID Controller for tracking speed : MATLAB Function  TreatAsAtomicUnit=on  SystemSampleTime=ts
  torque_cmd : Outport
  brake_cmd : Outport  Port=2
  wires:
  par/1 -> Bus Selector2/1, Bus Selector1/1
  Bus Selector1/1 -> PID Controller for tracking speed/4(ts)  "<ts>"
  Bus Selector1/2 -> PID Controller for tracking speed/5(max_drv_torque)  "<max_drv_torque>"
  Bus Selector1/3 -> PID Controller for tracking speed/6(max_delta_torque)  "<max_delta_torque>"
  Bus Selector1/4 -> PID Controller for tracking speed/7(min_brk_torque)  "<min_brk_torque>"
  Bus Selector1/5 -> PID Controller for tracking speed/8(max_delta_brake)  "<max_delta_brake>"
  Bus Selector1/6 -> PID Controller for tracking speed/9(kp)  "<kp_speed>"
  Bus Selector1/7 -> PID Controller for tracking speed/10(ki)  "<ki_speed>"
  Bus Selector1/8 -> PID Controller for tracking speed/11(kd)  "<kd_speed>"
  Bus Selector1/9 -> PID Controller for tracking speed/12(kff)  "<kff_gain>"
  Bus Selector1/10 -> PID Controller for tracking speed/13(fbreak_diff)  "<fbreak_diff>"
  Bus Selector1/11 -> PID Controller for tracking speed/14(fbreak_fflpf)  "<fbreak_fflpf>"
  verror/1 -> PID Controller for tracking speed/3(verror)  "velocity error"
  pitch/1 -> PID Controller for tracking speed/2(pitch)
  speed_mode/1 -> Compensate brake path/1(speed_mode), PID Controller for tracking speed/1(speed_mode)
  Bus Selector2/1 -> Compensate brake path/3(ts)  "<ts>"
  Bus Selector2/2 -> Compensate brake path/4(wT)  "<wT>"
  Bus Selector2/3 -> Compensate brake path/5(zT)  "<zT>"
  Bus Selector2/4 -> Compensate brake path/6(wB)  "<wB>"
  Bus Selector2/5 -> Compensate brake path/7(zB)  "<zB>"
  PID Controller for tracking speed/1(torque_cmd) -> Compensate brake path/2(torque_cmd)
  Compensate brake path/1(throttle_cmd) -> torque_cmd/1  "torque_cmd"
  Compensate brake path/2(brake_cmd) -> brake_cmd/1  "brake_cmd"
  Bus Selector2/6 -> Compensate brake path/8(min_brk_torque)  "<min_brk_torque>"

== system VC_v1p1/Vehicle_Controller/Longitudinal Control/Longitudinal Controller/velocity feedback pre-processor ==
  speed_mode : Inport
  vref : Inport  Port=2
  vcar : Inport  Port=3
  alat : Inport  Port=4
  along : Inport  Port=5
  par : Inport  Port=6
  Bus Selector1 : BusSelector  OutputSignals=ts,max_speed,max_alat,fbreak_vref,vdead
  MATLAB Function : MATLAB Function  TreatAsAtomicUnit=on  SystemSampleTime=ts
  Unit Delay : UnitDelay  SampleTime=ts  HasFrameUpgradeWarning=on
  vdes : Outport
  car_is_stopped : Outport  Port=2
  verror : Outport  Port=3
  wires:
  vref/1 -> MATLAB Function/2(vref)
  speed_mode/1 -> MATLAB Function/1(speed_mode)
  Bus Selector1/3 -> MATLAB Function/8(max_alat)  "<max_alat>"
  Bus Selector1/1 -> MATLAB Function/6(ts)  "<ts>"
  Bus Selector1/2 -> MATLAB Function/7(max_speed)  "<max_speed>"
  MATLAB Function/1(vdes) -> vdes/1  "vdes"
  alat/1 -> MATLAB Function/4(alat)
  Bus Selector1/4 -> MATLAB Function/9(fbreak_vref)  "<fbreak_vref>"
  par/1 -> Bus Selector1/1
  vcar/1 -> MATLAB Function/3(vcar)
  MATLAB Function/2(verror) -> verror/1
  Bus Selector1/5 -> MATLAB Function/10(vdead)  "<vdead>"
  along/1 -> Unit Delay/1
  MATLAB Function/3(car_is_stopped) -> car_is_stopped/1
  Unit Delay/1 -> MATLAB Function/5(along)

== system VC_v1p1/Vehicle_Controller/Waypoint Path Analyzer/Waypoint Path Analysis/Check for end-of-data ==
  waypoint_index : Inport
  WPT_BUS : Inport  Port=2
  Bus Selector1 : BusSelector  OutputSignals=NUM_WP
  Data Type Conversion : DataTypeConversion  OutDataTypeStr=double  SaturateOnIntegerOverflow=off  RndMeth=Floor
  Relational Operator : RelationalOperator  OutDataTypeStr=boolean  RndMeth=Simplest  InputSameDT=off
  end_of_data : Outport
  wires:
  WPT_BUS/1 -> Bus Selector1/1
  Bus Selector1/1 -> Relational Operator/2  "<NUM_WP>"
  waypoint_index/1 -> Relational Operator/1
  Relational Operator/1 -> Data Type Conversion/1
  Data Type Conversion/1 -> end_of_data/1

== system VC_v1p1/Vehicle_Controller/Waypoint Path Analyzer/Waypoint Path Analysis/Estimate closest point on path to vehicle ==
  path_mode : Inport
  northr : Inport  Port=2
  eastr : Inport  Port=3
  wpt_status_change : Inport  Port=4
  WPT_BUS : Inport  Port=5
  Bus Selector1 : BusSelector  OutputSignals=NUM_WP,NWP (m),EWP (m),VWP (m/s),SWP (bitfield)
  Estimate key parameters at closest path point : MATLAB Function  TreatAsAtomicUnit=on  SystemSampleTime=ts
  wpt_index : Outport
  northc : Outport  Port=2
  eastc : Outport  Port=3
  vref : Outport  Port=4
  signal_cmd : Outport  Port=5
  xterr : Outport  Port=6
  wires:
  Estimate key parameters at closest path point/1(wpt_index) -> wpt_index/1
  eastr/1 -> Estimate key parameters at closest path point/3(eastr)
  northr/1 -> Estimate key parameters at closest path point/2(northr)
  path_mode/1 -> Estimate key parameters at closest path point/1(path_mode)
  WPT_BUS/1 -> Bus Selector1/1
  Bus Selector1/1 -> Estimate key parameters at closest path point/5(NUM_WP)  "<NUM_WP>"
  Bus Selector1/2 -> Estimate key parameters at closest path point/6(NWP)  "<NWP (m)>"
  Bus Selector1/3 -> Estimate key parameters at closest path point/7(EWP)  "<EWP (m)>"
  Estimate key parameters at closest path point/2(north) -> northc/1
  Estimate key parameters at closest path point/3(east) -> eastc/1
  wpt_status_change/1 -> Estimate key parameters at closest path point/4(wpt_status_change)
  Bus Selector1/4 -> Estimate key parameters at closest path point/8(VWP)  "<VWP (m/s)>"
  Bus Selector1/5 -> Estimate key parameters at closest path point/9(SWP)  "<SWP (bitfield)>"
  Estimate key parameters at closest path point/4(vref) -> vref/1
  Estimate key parameters at closest path point/5(signal) -> signal_cmd/1
  Estimate key parameters at closest path point/6(xterr) -> xterr/1

== system VC_v1p1/Vehicle_Controller/Waypoint Path Analyzer/Waypoint Path Analysis/Estimate lookahead target point ==
  path_mode : Inport
  wpt_index : Inport  Port=2
  northc : Inport  Port=3
  eastc : Inport  Port=4
  par : Inport  Port=5
  WP_BUS : Inport  Port=6
  Bus Selector1 : BusSelector  OutputSignals=NUM_WP,NWP (m),EWP (m)
  Bus Selector2 : BusSelector  OutputSignals=min_lookahead,max_lookahead
  MATLAB Function : MATLAB Function  TreatAsAtomicUnit=on  SystemSampleTime=ts
  Terminator : Terminator
  northt : Outport
  eastt : Outport  Port=2
  wires:
  wpt_index/1 -> MATLAB Function/2(wpt_index)
  WP_BUS/1 -> Bus Selector1/1
  Bus Selector1/1 -> MATLAB Function/7(NUM_WP)  "<NUM_WP>"
  Bus Selector1/2 -> MATLAB Function/8(NWP)  "<NWP (m)>"
  Bus Selector1/3 -> MATLAB Function/9(EWP)  "<EWP (m)>"
  eastc/1 -> MATLAB Function/4(eastc)
  northc/1 -> MATLAB Function/3(northc)
  MATLAB Function/2(northt) -> northt/1
  MATLAB Function/3(eastt) -> eastt/1
  MATLAB Function/1(target_index) -> Terminator/1
  path_mode/1 -> MATLAB Function/1(path_mode)
  par/1 -> Bus Selector2/1
  Bus Selector2/1 -> MATLAB Function/5(minLA)  "<min_lookahead>"
  Bus Selector2/2 -> MATLAB Function/6(maxLA)  "<max_lookahead>"

== system VC_v1p1/Vehicle_Controller/Lateral Control/Lateral Controller/Calculate control limits/Calculate Target Distance ==
  note: Euclidean distance between Car and Target points
  Etarget : Inport
  Ecar : Inport  Port=2
  Ntarget : Inport  Port=3
  Ncar : Inport  Port=4
  Product : Product
  Product1 : Product
  Sqrt : Sqrt
  Sum : Sum  Inputs=|+-
  Sum1 : Sum  Inputs=|+-
  Sum2 : Sum  Inputs=+|+
  R : Outport
  wires:
  Sqrt/1 -> R/1  "distance"
  Ecar/1 -> Sum/2
  Etarget/1 -> Sum/1
  Ntarget/1 -> Sum1/1
  Sum2/1 -> Sqrt/1
  Product1/1 -> Sum2/2  "delta_N_squared"
  Product/1 -> Sum2/1  "delta_E_squared"
  Ncar/1 -> Sum1/2
  Sum/1 -> Product/2, Product/1  "delta_E"
  Sum1/1 -> Product1/2, Product1/1  "delta_N"

== system VC_v1p1/Vehicle_Controller/Lateral Control/Lateral Controller/Calculate control limits/Choose Conservative Curvature Rate Limits ==
  kpmax_spd : Inport
  kpmax_geo : Inport  Port=2
  kpmin_geo : Inport  Port=3
  Gain : Gain  Gain=-1
  Relational Operator : RelationalOperator  Operator=<  OutDataTypeStr=boolean  RndMeth=Simplest  InputSameDT=off
  Relational Operator1 : RelationalOperator  Operator=>  OutDataTypeStr=boolean  RndMeth=Simplest  InputSameDT=off
  Switch : Switch  Criteria=u2 > Threshold  SaturateOnIntegerOverflow=off  InputSameDT=off
  Switch1 : Switch  Criteria=u2 > Threshold  SaturateOnIntegerOverflow=off  InputSameDT=off
  kpmax : Outport
  kpmin : Outport  Port=2
  wires:
  Relational Operator/1 -> Switch/2
  kpmax_geo/1 -> Relational Operator/1, Switch/1  "kpmax_geo"
  kpmax_spd/1 -> Relational Operator/2, Switch/3, Gain/1  "kpmax_spd"
  Switch/1 -> kpmax/1
  Relational Operator1/1 -> Switch1/2
  Switch1/1 -> kpmin/1
  kpmin_geo/1 -> Relational Operator1/2, Switch1/3  "kpmin_geo"
  Gain/1 -> Switch1/1, Relational Operator1/1  "-kpmax_spd"

== stateflow chart VC_v1p1/Chevy Bolt EUV 2023 and GNSS/engine-steer-brake and inertial dynamics/Gear Change FSM ==
  state PARK
    en:  gear_fbk = 0;
  state DRIVE
    en:  gear_fbk = 1;
  state REVERSE
    en:  gear_fbk = -1;
  PARK -> PARK [order 3]
  (default) -> PARK
  PARK -> DRIVE [order 1] : [(gear_cmd==1) &&  ...
      | (abs(vcg) <= Vdead) && ...
      | (abs(brake_fbk) > Tdead)]
  DRIVE -> PARK [order 1] : [(gear_cmd==0) &&  ...
      | (abs(vcg) <= Vdead) && ...
      | (abs(brake_fbk) > Tdead)]
  REVERSE -> PARK [order 1] : [(gear_cmd==0) &&  ...
      | (abs(vcg) <= Vdead) && ...
      | (abs(brake_fbk) > Tdead)]
  PARK -> REVERSE [order 2] : [(gear_cmd==-1) &&  ...
      | (abs(vcg) <= Vdead) && ...
      | (abs(brake_fbk) > Tdead)]
  REVERSE -> REVERSE [order 3]
  DRIVE -> DRIVE [order 3]
  DRIVE -> REVERSE [order 2] : [(gear_cmd==-1) &&  ...
      | (abs(vcg) <= Vdead) && ...
      | (abs(brake_fbk) > Tdead)]
  REVERSE -> DRIVE [order 2] : [(gear_cmd==1) &&  ...
      | (abs(vcg) <= Vdead) && ...
      | (abs(brake_fbk) > Tdead)]
  data: gear_cmd input; vcg input; brake_fbk input; gear_fbk output; Tdead input; Vdead input

== stateflow chart VC_v1p1/Path Planner Emulator/Local Planner FSM ==
  state wait_for_autonomous_operation
    en:  action_select = 0;  % HOLDING_PATTERN
  state request_VC_ready_brake
    en:  action_select = 1;  % INIT_AUTO
  state request_VC_run_hot
    en:  action_select = 2;  % RUN_HOT
  (default) -> wait_for_autonomous_operation
  wait_for_autonomous_operation -> wait_for_autonomous_operation [order 2]
  request_VC_run_hot -> wait_for_autonomous_operation : [mode_select == 0]
  request_VC_ready_brake -> wait_for_autonomous_operation [order 1] : [mode_select == 0]
  wait_for_autonomous_operation -> request_VC_ready_brake [order 1] : [mode_select ~= 0]
  request_VC_ready_brake -> request_VC_ready_brake [order 3]
  request_VC_ready_brake -> request_VC_run_hot [order 2] : [VC_STATE == 2]
  data: mode_select input; action_select output; VC_STATE input

== matlab function VC_v1p1/Chevy Bolt EUV 2023 and GNSS/GNSS measurement/MATLAB Function ==
  data: x input; z output; y input
function z = vc_mod(x,y)
%
%  Alternative to the Matlab mod(x,y) function that does not require a
%  divide and can be converted to C or C++ properly.

%  Last Updated:  1/5/2023

%  --determine the sign of the input data
x_is_negative = false;
if ( x < 0 )
    %  --input x is negative
    x_is_negative = true;
    x = - x;
end


%  --find the interval n
n = 1;
while ( x >= n*y )
    n = n + 1;
end
n = n - 1;


%  --get the positive remainder
z = x - n*y;


%  --adjust for negative values
if ( x_is_negative )
    if ( x == n*y )
        z = - z;
    else
        z = y - z;
    end
end

== stateflow chart VC_v1p1/Vehicle_Controller/Operational State Machine/VC_FSM ==
  state MANUAL_S0
    en:  VC_state = 0;
    en:  AV_start_request = 0;
    en:  speed_mode = 0;
    en:  steer_mode = 0;
    en:  path_mode = 0;
    en:  counter = 0;
  state INIT_AUTO_S1
    en:  VC_state = 1;
    en:  path_mode = 0;
    en:  AV_start_request = 1;
    en: if ((mode_select == 1) || (mode_select == 2))
    % autonomous speed control
    speed_mode = 0; % zero torque and brake
    end
    en:  if ((mode_select == 1) || (mode_select == 3))
    % autonomous steer control
    steer_mode = 0; % zero steer command
    end
  note: mode_select
      | 0 = manual
      | 1 = full autonomous
      | 2 = autonomous speed
      | 3 = autonomous steer
      |
      | action_select
      | 0 = enter manual mode
      | 1 = enter autonomous mode
      | 2 = enter run_hot mode
      |
      | speed_mode
      | 0 = zero torque and brake commands
      | 1 = max brake and zero torque
      | 2 = internal commands
      |
      | steer_mode
      | 0 = zero steer command
      | 1 = hold steering command at current value
      | 2 = internal command
      |
      | path_mode
      | 0 = disable analysis
      | 1 = enable analysis
  state RDY_BRAKE_S2
    en:  VC_state = 2;
    en:  path_mode = 1;
    en:  AV_start_request = 1;
    en:  if ((mode_select == 1) || (mode_select == 2))
    % autonomous speed control
    speed_mode = 1; % max brake, zero torque
    end
    en:  if ((mode_select == 1) || (mode_select == 3))
    % autonomous steer control
    steer_mode = 1; % hold steering command
    end
    du:  if (counter > 100), counter = 0; end
  state RUN_HOT_S3
    en:  VC_state = 3;
    en:  AV_start_request = 1;
    en:  path_mode = 1;
    en:  if ((mode_select == 1) || (mode_select == 2))
    % autonomous speed control
    speed_mode = 2; % internal
    end
    en:  if ((mode_select == 1) || (mode_select == 3))
    % autonomous steer control
    steer_mode = 2; % internal
    end
  (default) -> MANUAL_S0
  MANUAL_S0 -> MANUAL_S0 [order 2]
  (junction 50) -> MANUAL_S0
  (junction 48) -> (junction 50)
  MANUAL_S0 -> INIT_AUTO_S1 [order 1] : [(mode_select > 0) & ...
      |  (action_select == 1) & ...
      | (car_is_stopped == 1)]
  INIT_AUTO_S1 -> INIT_AUTO_S1 [order 3]
  INIT_AUTO_S1 -> (junction 48) [order 1] : [(mode_select == 0) || ...
      | (action_select == 0)]
  (junction 53) -> (junction 48)
  INIT_AUTO_S1 -> RDY_BRAKE_S2 [order 2] : [(AV_mode_active == 1) & ...
      | (action_select == 1)]
  RDY_BRAKE_S2 -> RDY_BRAKE_S2 [order 3] : [action_select ~= 0] ...
      | {counter = counter + 1;}
  RDY_BRAKE_S2 -> (junction 53) [order 1] : [(mode_select == 0) || ...
      | (action_select == 0) || ...
      | (AV_mode_active == 0)]
  (junction 57) -> (junction 53)
  RDY_BRAKE_S2 -> RUN_HOT_S3 [order 2] : [(action_select == 2) & ...
      | (counter >= 100)]
  RUN_HOT_S3 -> RDY_BRAKE_S2 [order 2] : [(car_is_stopped == 1) & ...
      | (end_of_data == 1)]
  RUN_HOT_S3 -> RUN_HOT_S3 [order 3]
  RUN_HOT_S3 -> (junction 57) [order 1] : [(mode_select == 0) || ...
      | (action_select == 0) || ...
      | (AV_mode_active == 0)]
  data: VC_state output; speed_mode output; steer_mode output; mode_select input; action_select input; car_is_stopped input; path_mode output; AV_mode_active input; AV_start_request output; end_of_data input; counter local
